simulink subsystem "s0330_swing_up_controller"  (R2019b)
settings: Solver=VariableStepAuto  StartTime=0.0  StopTime=10.0  RelTol=1e-3
undefined symbols (not defined in the file): __PRM__SERIALIZED__DATA__, PARAMS, SubsystemReferenceBlock
settings Model: Creator=paolo  LastModifiedBy=giaco

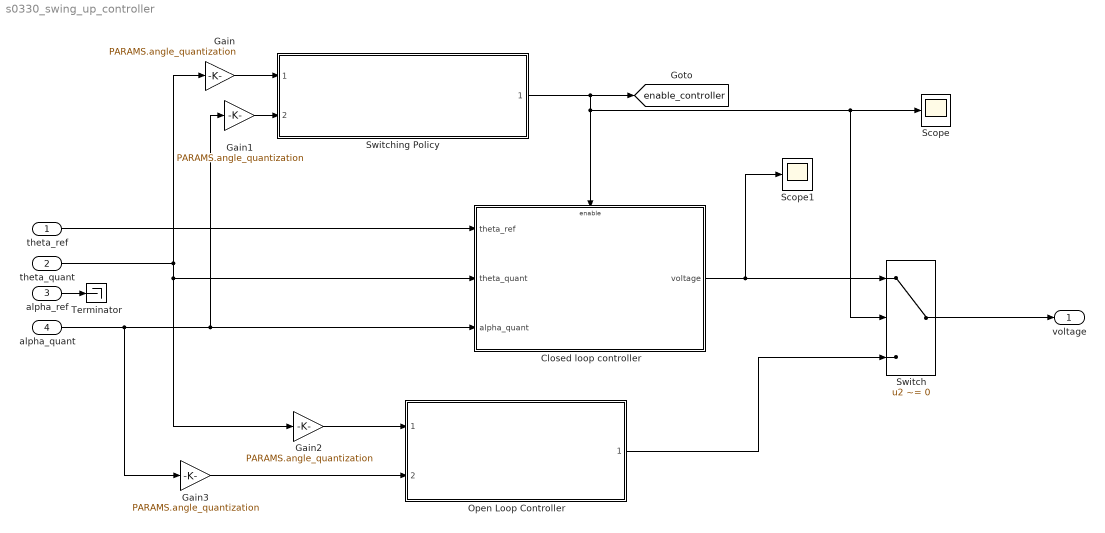
== system s0330_swing_up_controller ==
  theta_ref : Inport
  theta_quant : Inport  Port=2
  alpha_ref : Inport  Port=3
  alpha_quant : Inport  Port=4
  Closed loop controller : Subsystem
  Gain{,1..3} (4 alike) : Gain  Gain=PARAMS.angle_quantization
  Open Loop Controller : Subsystem  BlockKeywords=__PRM__SERIALIZED__DATA__:SubsystemReferenceBlock  ReferencedSubsystem=s0411_swing_fast2
  Scope : Scope
  Scope1 : Scope
  Switch : Switch  Criteria=u2 ~= 0
  Switching Policy : Subsystem  BlockKeywords=__PRM__SERIALIZED__DATA__:SubsystemReferenceBlock  ReferencedSubsystem=s0518_switching_policy3
  Terminator : Terminator
  voltage : Outport
  tag scope: enable_controller=global
  wires:
  alpha_quant/1 -> Gain3/1, Closed loop controller/3(alpha_quant), Gain1/1
  Switch/1 -> voltage/1
  Open Loop Controller/1 -> Switch/3
  alpha_ref/1 -> Terminator/1
  theta_quant/1 -> Gain2/1, Closed loop controller/2(theta_quant), Gain/1
  theta_ref/1 -> Closed loop controller/1(theta_ref)
  Closed loop controller/1(voltage) -> Switch/1, Scope1/1
  Switching Policy/1 -> [enable_controller], Closed loop controller/Enable, Scope/1, Switch/2
  Gain/1 -> Switching Policy/1
  Gain1/1 -> Switching Policy/2
  Gain2/1 -> Open Loop Controller/1
  Gain3/1 -> Open Loop Controller/2

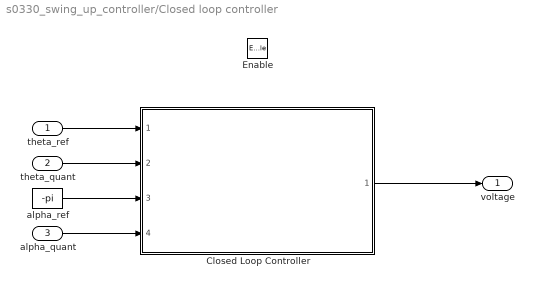
== system s0330_swing_up_controller/Closed loop controller ==
  theta_ref : Inport
  theta_quant : Inport  Port=2
  alpha_quant : Inport  Port=3
  Enable : EnablePort  StatesWhenEnabling=reset
  Closed Loop Controller : Subsystem  BlockKeywords=__PRM__SERIALIZED__DATA__:SubsystemReferenceBlock  ReferencedSubsystem=s0320_alpha_theta_PP
  "alpha_ref " : Constant  Value=-pi
  voltage : Outport
  wires:
  Closed Loop Controller/1 -> voltage/1
  theta_ref/1 -> Closed Loop Controller/1
  "alpha_ref "/1 -> Closed Loop Controller/3
  alpha_quant/1 -> Closed Loop Controller/4
  theta_quant/1 -> Closed Loop Controller/2
